simulink model "SAS"  (R2017b)
settings: Solver=VariableStepAuto  StartTime=0.0  StopTime=10.0  RelTol=1e-3
values from neighbouring files (symbols this model uses):
  A = A'    [c_l.m]    (also in c_m.m; c_n.m; c_x.m; c_z.m)
  altitude = input('Enter the altitude for the simulation (ft)  :  ')    [FindF16Dynamics.m]    (also in run_me.m = input(' altitude ( 0 ~ 40000 ft ) : '); trim_F16.m = alt)
  B = ssm_b( state_trim, state_dot_trim, control_trim, xcg )    [ssm_f16.m]    (also in thrust.m = B')
  C = ssm_c( state_trim, state_dot_trim, control_trim, xcg )    [ssm_f16.m]    (also in thrust.m = C')
  C_1 = eye(10)    [run_me.m]
  control_trim = u0    [find_trim.m]
  D = ssm_d( state_trim, state_dot_trim, control_trim, xcg )    [ssm_f16.m]
  D_1 = zeros(10,4)    [run_me.m]
  state_trim = steady_state( state )    [find_trim.m]
  velocity = input('Enter the velocity for the simulation (ft/s):  ')    [FindF16Dynamics.m]    (also in run_me.m = input(' true velocity ( 350 ~ 1000 ft/sec ) : '); trim_F16.m = vel)
libraries: simulink x7
settings Model: Creator=monster  LastModifiedBy=monster

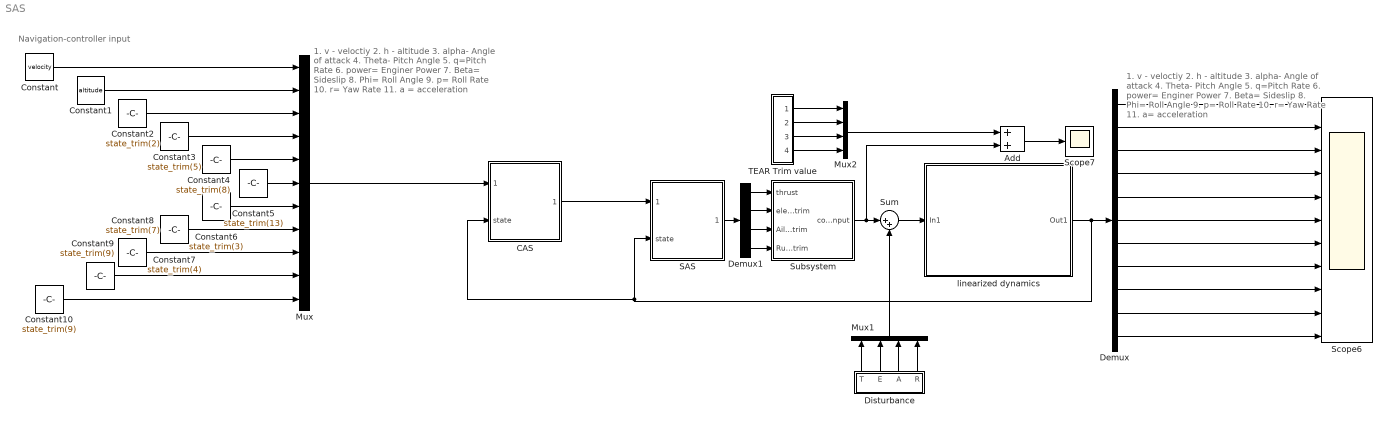
== system SAS ==
  note: Navigation-controller input
  note: 1. v - veloctiy
      |
      | 2. h - altitude
      |
      | 3. alpha- Angle of attack
      |
      | 4. Theta- Pitch Angle
      |
      | 5. q=Pitch Rate
      |
      | 6. power= Enginer Power
      |
      | 7. Beta= Sideslip
      |
      | 8. Phi= Roll Angle
      |
      | 9. p= Roll Rate
      |
      | 10. r= Yaw Rate
      |
      | 11. a= acceleration
  note: 1. v - veloctiy
      |
      | 2. h - altitude
      |
      | 3. alpha- Angle of attack
      |
      | 4. Theta- Pitch Angle
      |
      | 5. q=Pitch Rate
      |
      | 6. power= Enginer Power
      |
      | 7. Beta= Sideslip
      |
      | 8. Phi= Roll Angle
      |
      | 9. p= Roll Rate
      |
      | 10. r= Yaw Rate
      |
      | 11. a = acceleration
  " Disturbance" : Subsystem
  Add : Sum
  CAS : Subsystem
  Constant : Constant  Value=velocity
  Constant1 : Constant  Value=altitude
  Constant10 : Constant  Value=state_trim(9)
  Constant2 : Constant  Value=state_trim(2)
  Constant3 : Constant  Value=state_trim(5)
  Constant4 : Constant  Value=state_trim(8)
  Constant5 : Constant  Value=state_trim(13)
  Constant6 : Constant  Value=state_trim(3)
  Constant7 : Constant  Value=state_trim(4)
  Constant8 : Constant  Value=state_trim(7)
  Constant9 : Constant  Value=state_trim(9)
  Demux : Demux  Outputs=11
  Demux1 : Demux
  Mux : Mux  Inputs=11
  Mux1 : Mux
  Mux2 : Mux
  SAS : Subsystem
  Scope6 : Scope  NumInputPorts=11
  Scope7 : Scope
  Subsystem : Subsystem
  Sum : Sum  Inputs=|++
  "TEAR Trim value " : Subsystem
  linearized dynamics : Subsystem
      mask Display: image('D:\Dropbox\M.eng\fall2017\flight control system\FDC\project\control surface.PNG');
  wires:
  Demux/10 -> Scope6/10
  Subsystem/1(control_input) -> Sum/1, Add/2
  Demux1/1 -> Subsystem/1(thrust)
  Demux1/2 -> Subsystem/2(elevator_trim)
  Demux1/3 -> Subsystem/3(Aileron_trim)
  "TEAR Trim value "/4(R) -> Mux2/4
  Demux/6 -> Scope6/6
  Demux1/4 -> Subsystem/4(Rudder_trim)
  "TEAR Trim value "/1(T) -> Mux2/1
  Demux/7 -> Scope6/7
  "TEAR Trim value "/2(E) -> Mux2/2
  Demux/2 -> Scope6/2
  Add/1 -> Scope7/1
  Demux/4 -> Scope6/4
  Demux/3 -> Scope6/3
  Demux/8 -> Scope6/8
  "TEAR Trim value "/3(A) -> Mux2/3
  Mux2/1 -> Add/1
  Demux/1 -> Scope6/1
  Demux/5 -> Scope6/5
  Demux/9 -> Scope6/9
  SAS/1(control_input) -> Demux1/1
  Mux/1 -> CAS/1(reference)
  Constant7/1 -> Mux/8
  Constant5/1 -> Mux/6
  Constant8/1 -> Mux/9
  Constant9/1 -> Mux/10
  Constant/1 -> Mux/1
  Constant4/1 -> Mux/5
  Constant3/1 -> Mux/4
  Constant2/1 -> Mux/3
  Constant6/1 -> Mux/7
  Constant1/1 -> Mux/2
  linearized dynamics/1(Out1) -> CAS/2(state), SAS/2(state), Demux/1
  Demux/11 -> Scope6/11
  Constant10/1 -> Mux/11
  Sum/1 -> linearized dynamics/1(In1)
  " Disturbance"/4(R) -> Mux1/4
  " Disturbance"/1(T) -> Mux1/1
  " Disturbance"/3(A) -> Mux1/3
  " Disturbance"/2(E) -> Mux1/2
  Mux1/1 -> Sum/2
  CAS/1(control_input) -> SAS/1(reference)

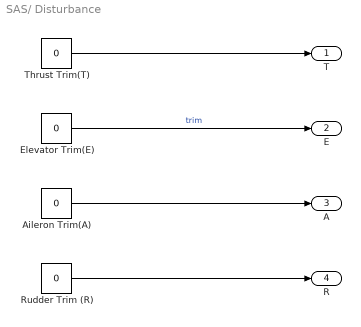
== system SAS/ Disturbance ==
  "Aileron Trim(A) " : Constant  Value=0
  "Elevator Trim(E) " : Constant  Value=0  VectorParams1D=off
  Rudder Trim (R) : Constant  Value=0
  "Thrust Trim(T) " : Constant  Value=0
  T : Outport
  E : Outport  Port=2
  A : Outport  Port=3
  R : Outport  Port=4
  wires:
  "Aileron Trim(A) "/1 -> A/1
  "Elevator Trim(E) "/1 -> E/1  "trim"
  "Thrust Trim(T) "/1 -> T/1
  Rudder Trim (R)/1 -> R/1

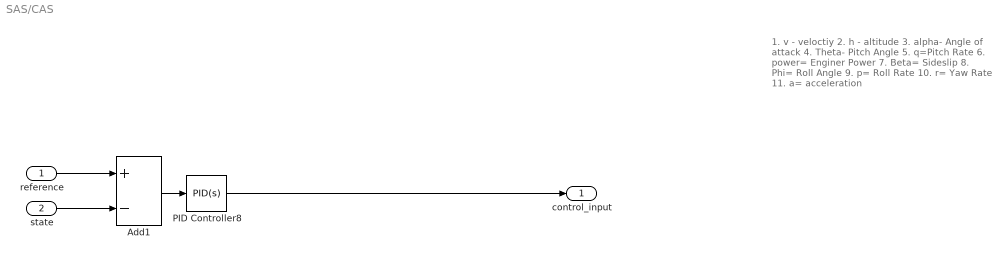
== system SAS/CAS ==
  note: 1. v - veloctiy
      |
      | 2. h - altitude
      |
      | 3. alpha- Angle of attack
      |
      | 4. Theta- Pitch Angle
      |
      | 5. q=Pitch Rate
      |
      | 6. power= Enginer Power
      |
      | 7. Beta= Sideslip
      |
      | 8. Phi= Roll Angle
      |
      | 9. p= Roll Rate
      |
      | 10. r= Yaw Rate
      |
      | 11. a= acceleration
  reference : Inport
  state : Inport  Port=2
  Add1 : Sum  Inputs=+-
  PID Controller8 : simulink/Continuous/PID Controller  Controller=PID  TimeDomain=Continuous-time  SampleTime=-1  IntegratorMethod=Forward Euler  FilterMethod=Forward Euler  Form=Parallel  UseFilter=on  ControllerParametersSource=internal  P=-49327.5398646116  I=-459229.123376859  D=-1288.80480278299  N=1181.77739704053  InitialConditionSource=internal  InitialConditionForIntegrator=0  InitialConditionForFilter=0  ExternalReset=none  LimitOutput=off  UpperSaturationLimit=inf  LowerSaturationLimit=-inf  LinearizeAsGain=on  AntiWindupMode=none  Kb=1  TrackingMode=off  Kt=1  PParamMin=[]  PParamMax=[]  IParamMin=[]  IParamMax=[]  DParamMin=[]  DParamMax=[]  NParamMin=[]  NParamMax=[]  KbParamMin=[]  KbParamMax=[]  KtParamMin=[]  KtParamMax=[]  POutMin=[]  POutMax=[]  IOutMin=[]  IOutMax=[]  DOutMin=[]  DOutMax=[]  NOutMin=[]  NOutMax=[]  KbOutMin=[]  KbOutMax=[]  KtOutMin=[]  KtOutMax=[]  IntegratorOutMin=[]  IntegratorOutMax=[]  FilterOutMin=[]  FilterOutMax=[]  SumOutMin=[]  SumOutMax=[]  SumI1OutMin=[]  SumI1OutMax=[]  SumI2OutMin=[]  SumI2OutMax=[]  SumI3OutMin=[]  SumI3OutMax=[]  SumDOutMin=[]  SumDOutMax=[]  SaturationOutMin=[]  SaturationOutMax=[]  IntegratorContinuousStateAttributes=''  IntegratorStateMustResolveToSignalObject=off  IntegratorRTWStateStorageClass=Auto  FilterContinuousStateAttributes=''  FilterStateMustResolveToSignalObject=off  FilterRTWStateStorageClass=Auto  DifferentiatorICPrevScaledInput=0  DifferentiatorOutMin=[]  DifferentiatorOutMax=[]  InitialConditionSetting=State (most efficient)  FilterDiffOutCoefMin=[]  FilterDiffOutCoefMax=[]  SumDenOutMin=[]  SumDenOutMax=[]  SumNumOutMin=[]  SumNumOutMax=[]  ReciprocalOutMin=[]  ReciprocalOutMax=[]  DivideOutMin=[]  DivideOutMax=[]  TunerSelectOption=Transfer Function Based (PID Tuner App)
  control_input : Outport
  wires:
  PID Controller8/1 -> control_input/1
  Add1/1 -> PID Controller8/1
  reference/1 -> Add1/1
  state/1 -> Add1/2

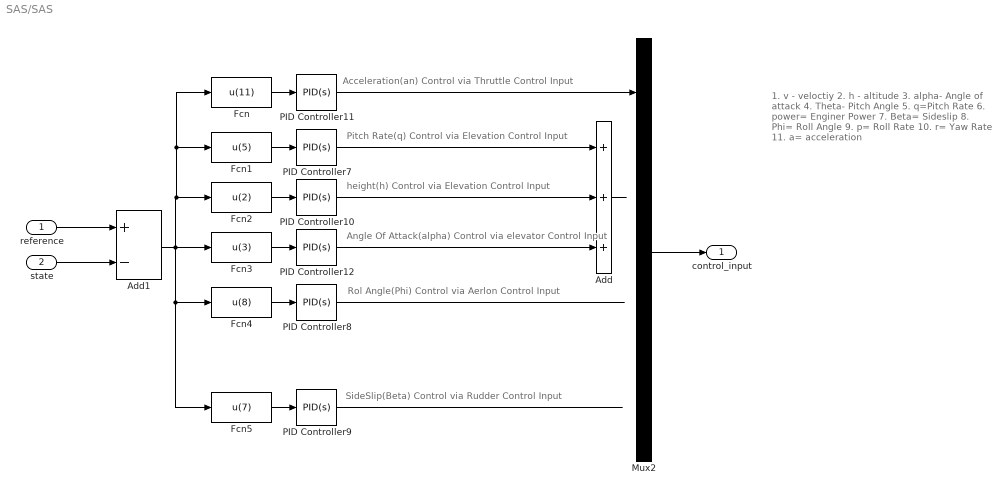
== system SAS/SAS ==
  note: Rol Angle(Phi) Control via Aerlon Control Input
  note: height(h) Control via Elevation Control Input
  note: Pitch Rate(q) Control via Elevation Control Input
  note: Acceleration(an) Control via Thruttle Control Input
  note: Angle Of Attack(alpha) Control via elevator Control Input
  note: SideSlip(Beta) Control via Rudder Control Input
  note: 1. v - veloctiy
      |
      | 2. h - altitude
      |
      | 3. alpha- Angle of attack
      |
      | 4. Theta- Pitch Angle
      |
      | 5. q=Pitch Rate
      |
      | 6. power= Enginer Power
      |
      | 7. Beta= Sideslip
      |
      | 8. Phi= Roll Angle
      |
      | 9. p= Roll Rate
      |
      | 10. r= Yaw Rate
      |
      | 11. a= acceleration
  reference : Inport
  state : Inport  Port=2
  Add : Sum  Inputs=+++
  Add1 : Sum  Inputs=+-
  Fcn : Fcn  Expr=u(11)
  Fcn1 : Fcn  Expr=u(5)
  Fcn2 : Fcn  Expr=u(2)
  Fcn3 : Fcn  Expr=u(3)
  Fcn4 : Fcn  Expr=u(8)
  Fcn5 : Fcn  Expr=u(7)
  Mux2 : Mux
  PID Controller10 : simulink/Continuous/PID Controller  Controller=PID  TimeDomain=Continuous-time  SampleTime=-1  IntegratorMethod=Forward Euler  FilterMethod=Forward Euler  Form=Parallel  UseFilter=on  ControllerParametersSource=internal  P=24508600.1259152  I=4501969741.89748  D=28958.3047379278  N=690409.793644926  InitialConditionSource=internal  InitialConditionForIntegrator=0  InitialConditionForFilter=0  ExternalReset=none  LimitOutput=off  UpperSaturationLimit=inf  LowerSaturationLimit=-inf  LinearizeAsGain=on  AntiWindupMode=none  Kb=1  TrackingMode=off  Kt=1  PParamMin=[]  PParamMax=[]  IParamMin=[]  IParamMax=[]  DParamMin=[]  DParamMax=[]  NParamMin=[]  NParamMax=[]  KbParamMin=[]  KbParamMax=[]  KtParamMin=[]  KtParamMax=[]  POutMin=[]  POutMax=[]  IOutMin=[]  IOutMax=[]  DOutMin=[]  DOutMax=[]  NOutMin=[]  NOutMax=[]  KbOutMin=[]  KbOutMax=[]  KtOutMin=[]  KtOutMax=[]  IntegratorOutMin=[]  IntegratorOutMax=[]  FilterOutMin=[]  FilterOutMax=[]  SumOutMin=[]  SumOutMax=[]  SumI1OutMin=[]  SumI1OutMax=[]  SumI2OutMin=[]  SumI2OutMax=[]  SumI3OutMin=[]  SumI3OutMax=[]  SumDOutMin=[]  SumDOutMax=[]  SaturationOutMin=[]  SaturationOutMax=[]  IntegratorContinuousStateAttributes=''  IntegratorStateMustResolveToSignalObject=off  IntegratorRTWStateStorageClass=Auto  FilterContinuousStateAttributes=''  FilterStateMustResolveToSignalObject=off  FilterRTWStateStorageClass=Auto  DifferentiatorICPrevScaledInput=0  DifferentiatorOutMin=[]  DifferentiatorOutMax=[]  InitialConditionSetting=State (most efficient)  FilterDiffOutCoefMin=[]  FilterDiffOutCoefMax=[]  SumDenOutMin=[]  SumDenOutMax=[]  SumNumOutMin=[]  SumNumOutMax=[]  ReciprocalOutMin=[]  ReciprocalOutMax=[]  DivideOutMin=[]  DivideOutMax=[]  TunerSelectOption=Transfer Function Based (PID Tuner App)
  PID Controller11 : simulink/Continuous/PID Controller  Controller=PID  TimeDomain=Continuous-time  SampleTime=-1  IntegratorMethod=Forward Euler  FilterMethod=Forward Euler  Form=Parallel  UseFilter=on  ControllerParametersSource=internal  P=13329483.1324469  I=392847306.175743  D=98980.5300334758  N=109037.560099343  InitialConditionSource=internal  InitialConditionForIntegrator=0  InitialConditionForFilter=0  ExternalReset=none  LimitOutput=off  UpperSaturationLimit=inf  LowerSaturationLimit=-inf  LinearizeAsGain=on  AntiWindupMode=none  Kb=1  TrackingMode=off  Kt=1  PParamMin=[]  PParamMax=[]  IParamMin=[]  IParamMax=[]  DParamMin=[]  DParamMax=[]  NParamMin=[]  NParamMax=[]  KbParamMin=[]  KbParamMax=[]  KtParamMin=[]  KtParamMax=[]  POutMin=[]  POutMax=[]  IOutMin=[]  IOutMax=[]  DOutMin=[]  DOutMax=[]  NOutMin=[]  NOutMax=[]  KbOutMin=[]  KbOutMax=[]  KtOutMin=[]  KtOutMax=[]  IntegratorOutMin=[]  IntegratorOutMax=[]  FilterOutMin=[]  FilterOutMax=[]  SumOutMin=[]  SumOutMax=[]  SumI1OutMin=[]  SumI1OutMax=[]  SumI2OutMin=[]  SumI2OutMax=[]  SumI3OutMin=[]  SumI3OutMax=[]  SumDOutMin=[]  SumDOutMax=[]  SaturationOutMin=[]  SaturationOutMax=[]  IntegratorContinuousStateAttributes=''  IntegratorStateMustResolveToSignalObject=off  IntegratorRTWStateStorageClass=Auto  FilterContinuousStateAttributes=''  FilterStateMustResolveToSignalObject=off  FilterRTWStateStorageClass=Auto  DifferentiatorICPrevScaledInput=0  DifferentiatorOutMin=[]  DifferentiatorOutMax=[]  InitialConditionSetting=State (most efficient)  FilterDiffOutCoefMin=[]  FilterDiffOutCoefMax=[]  SumDenOutMin=[]  SumDenOutMax=[]  SumNumOutMin=[]  SumNumOutMax=[]  ReciprocalOutMin=[]  ReciprocalOutMax=[]  DivideOutMin=[]  DivideOutMax=[]  TunerSelectOption=Transfer Function Based (PID Tuner App)
  PID Controller12 : simulink/Continuous/PID Controller  Controller=PID  TimeDomain=Continuous-time  SampleTime=-1  IntegratorMethod=Forward Euler  FilterMethod=Forward Euler  Form=Parallel  UseFilter=on  ControllerParametersSource=internal  P=-170.14183467408  I=-465.695324804371  D=-13.6839697818054  N=105.697856042613  InitialConditionSource=internal  InitialConditionForIntegrator=0  InitialConditionForFilter=0  ExternalReset=none  LimitOutput=off  UpperSaturationLimit=inf  LowerSaturationLimit=-inf  LinearizeAsGain=on  AntiWindupMode=none  Kb=1  TrackingMode=off  Kt=1  PParamMin=[]  PParamMax=[]  IParamMin=[]  IParamMax=[]  DParamMin=[]  DParamMax=[]  NParamMin=[]  NParamMax=[]  KbParamMin=[]  KbParamMax=[]  KtParamMin=[]  KtParamMax=[]  POutMin=[]  POutMax=[]  IOutMin=[]  IOutMax=[]  DOutMin=[]  DOutMax=[]  NOutMin=[]  NOutMax=[]  KbOutMin=[]  KbOutMax=[]  KtOutMin=[]  KtOutMax=[]  IntegratorOutMin=[]  IntegratorOutMax=[]  FilterOutMin=[]  FilterOutMax=[]  SumOutMin=[]  SumOutMax=[]  SumI1OutMin=[]  SumI1OutMax=[]  SumI2OutMin=[]  SumI2OutMax=[]  SumI3OutMin=[]  SumI3OutMax=[]  SumDOutMin=[]  SumDOutMax=[]  SaturationOutMin=[]  SaturationOutMax=[]  IntegratorContinuousStateAttributes=''  IntegratorStateMustResolveToSignalObject=off  IntegratorRTWStateStorageClass=Auto  FilterContinuousStateAttributes=''  FilterStateMustResolveToSignalObject=off  FilterRTWStateStorageClass=Auto  DifferentiatorICPrevScaledInput=0  DifferentiatorOutMin=[]  DifferentiatorOutMax=[]  InitialConditionSetting=State (most efficient)  FilterDiffOutCoefMin=[]  FilterDiffOutCoefMax=[]  SumDenOutMin=[]  SumDenOutMax=[]  SumNumOutMin=[]  SumNumOutMax=[]  ReciprocalOutMin=[]  ReciprocalOutMax=[]  DivideOutMin=[]  DivideOutMax=[]  TunerSelectOption=Transfer Function Based (PID Tuner App)
  PID Controller7 : simulink/Continuous/PID Controller  Controller=PID  TimeDomain=Continuous-time  SampleTime=-1  IntegratorMethod=Forward Euler  FilterMethod=Forward Euler  Form=Parallel  UseFilter=on  ControllerParametersSource=internal  P=-2409.99420452658  I=-41171.6281036838  D=-4.63151383685818  N=352.425457454863  InitialConditionSource=internal  InitialConditionForIntegrator=0  InitialConditionForFilter=0  ExternalReset=none  LimitOutput=off  UpperSaturationLimit=inf  LowerSaturationLimit=-inf  LinearizeAsGain=on  AntiWindupMode=none  Kb=1  TrackingMode=off  Kt=1  PParamMin=[]  PParamMax=[]  IParamMin=[]  IParamMax=[]  DParamMin=[]  DParamMax=[]  NParamMin=[]  NParamMax=[]  KbParamMin=[]  KbParamMax=[]  KtParamMin=[]  KtParamMax=[]  POutMin=[]  POutMax=[]  IOutMin=[]  IOutMax=[]  DOutMin=[]  DOutMax=[]  NOutMin=[]  NOutMax=[]  KbOutMin=[]  KbOutMax=[]  KtOutMin=[]  KtOutMax=[]  IntegratorOutMin=[]  IntegratorOutMax=[]  FilterOutMin=[]  FilterOutMax=[]  SumOutMin=[]  SumOutMax=[]  SumI1OutMin=[]  SumI1OutMax=[]  SumI2OutMin=[]  SumI2OutMax=[]  SumI3OutMin=[]  SumI3OutMax=[]  SumDOutMin=[]  SumDOutMax=[]  SaturationOutMin=[]  SaturationOutMax=[]  IntegratorContinuousStateAttributes=''  IntegratorStateMustResolveToSignalObject=off  IntegratorRTWStateStorageClass=Auto  FilterContinuousStateAttributes=''  FilterStateMustResolveToSignalObject=off  FilterRTWStateStorageClass=Auto  DifferentiatorICPrevScaledInput=0  DifferentiatorOutMin=[]  DifferentiatorOutMax=[]  InitialConditionSetting=State (most efficient)  FilterDiffOutCoefMin=[]  FilterDiffOutCoefMax=[]  SumDenOutMin=[]  SumDenOutMax=[]  SumNumOutMin=[]  SumNumOutMax=[]  ReciprocalOutMin=[]  ReciprocalOutMax=[]  DivideOutMin=[]  DivideOutMax=[]  TunerSelectOption=Transfer Function Based (PID Tuner App)
  PID Controller8 : simulink/Continuous/PID Controller  Controller=PID  TimeDomain=Continuous-time  SampleTime=-1  IntegratorMethod=Forward Euler  FilterMethod=Forward Euler  Form=Parallel  UseFilter=on  ControllerParametersSource=internal  P=-49327.5398646116  I=-459229.123376859  D=-1288.80480278299  N=1181.77739704053  InitialConditionSource=internal  InitialConditionForIntegrator=0  InitialConditionForFilter=0  ExternalReset=none  LimitOutput=off  UpperSaturationLimit=inf  LowerSaturationLimit=-inf  LinearizeAsGain=on  AntiWindupMode=none  Kb=1  TrackingMode=off  Kt=1  PParamMin=[]  PParamMax=[]  IParamMin=[]  IParamMax=[]  DParamMin=[]  DParamMax=[]  NParamMin=[]  NParamMax=[]  KbParamMin=[]  KbParamMax=[]  KtParamMin=[]  KtParamMax=[]  POutMin=[]  POutMax=[]  IOutMin=[]  IOutMax=[]  DOutMin=[]  DOutMax=[]  NOutMin=[]  NOutMax=[]  KbOutMin=[]  KbOutMax=[]  KtOutMin=[]  KtOutMax=[]  IntegratorOutMin=[]  IntegratorOutMax=[]  FilterOutMin=[]  FilterOutMax=[]  SumOutMin=[]  SumOutMax=[]  SumI1OutMin=[]  SumI1OutMax=[]  SumI2OutMin=[]  SumI2OutMax=[]  SumI3OutMin=[]  SumI3OutMax=[]  SumDOutMin=[]  SumDOutMax=[]  SaturationOutMin=[]  SaturationOutMax=[]  IntegratorContinuousStateAttributes=''  IntegratorStateMustResolveToSignalObject=off  IntegratorRTWStateStorageClass=Auto  FilterContinuousStateAttributes=''  FilterStateMustResolveToSignalObject=off  FilterRTWStateStorageClass=Auto  DifferentiatorICPrevScaledInput=0  DifferentiatorOutMin=[]  DifferentiatorOutMax=[]  InitialConditionSetting=State (most efficient)  FilterDiffOutCoefMin=[]  FilterDiffOutCoefMax=[]  SumDenOutMin=[]  SumDenOutMax=[]  SumNumOutMin=[]  SumNumOutMax=[]  ReciprocalOutMin=[]  ReciprocalOutMax=[]  DivideOutMin=[]  DivideOutMax=[]  TunerSelectOption=Transfer Function Based (PID Tuner App)
  PID Controller9 : simulink/Continuous/PID Controller  Controller=PID  TimeDomain=Continuous-time  SampleTime=-1  IntegratorMethod=Forward Euler  FilterMethod=Forward Euler  Form=Parallel  UseFilter=on  ControllerParametersSource=internal  P=908.491475757153  I=143.160579860217  D=1280.97081759687  N=3086.89831654681  InitialConditionSource=internal  InitialConditionForIntegrator=0  InitialConditionForFilter=0  ExternalReset=none  LimitOutput=off  UpperSaturationLimit=inf  LowerSaturationLimit=-inf  LinearizeAsGain=on  AntiWindupMode=none  Kb=1  TrackingMode=off  Kt=1  PParamMin=[]  PParamMax=[]  IParamMin=[]  IParamMax=[]  DParamMin=[]  DParamMax=[]  NParamMin=[]  NParamMax=[]  KbParamMin=[]  KbParamMax=[]  KtParamMin=[]  KtParamMax=[]  POutMin=[]  POutMax=[]  IOutMin=[]  IOutMax=[]  DOutMin=[]  DOutMax=[]  NOutMin=[]  NOutMax=[]  KbOutMin=[]  KbOutMax=[]  KtOutMin=[]  KtOutMax=[]  IntegratorOutMin=[]  IntegratorOutMax=[]  FilterOutMin=[]  FilterOutMax=[]  SumOutMin=[]  SumOutMax=[]  SumI1OutMin=[]  SumI1OutMax=[]  SumI2OutMin=[]  SumI2OutMax=[]  SumI3OutMin=[]  SumI3OutMax=[]  SumDOutMin=[]  SumDOutMax=[]  SaturationOutMin=[]  SaturationOutMax=[]  IntegratorContinuousStateAttributes=''  IntegratorStateMustResolveToSignalObject=off  IntegratorRTWStateStorageClass=Auto  FilterContinuousStateAttributes=''  FilterStateMustResolveToSignalObject=off  FilterRTWStateStorageClass=Auto  DifferentiatorICPrevScaledInput=0  DifferentiatorOutMin=[]  DifferentiatorOutMax=[]  InitialConditionSetting=State (most efficient)  FilterDiffOutCoefMin=[]  FilterDiffOutCoefMax=[]  SumDenOutMin=[]  SumDenOutMax=[]  SumNumOutMin=[]  SumNumOutMax=[]  ReciprocalOutMin=[]  ReciprocalOutMax=[]  DivideOutMin=[]  DivideOutMax=[]  TunerSelectOption=Transfer Function Based (PID Tuner App)
  control_input : Outport
  wires:
  Mux2/1 -> control_input/1
  PID Controller11/1 -> Mux2/1
  Fcn5/1 -> PID Controller9/1
  Fcn3/1 -> PID Controller12/1
  PID Controller7/1 -> Add/1
  Fcn2/1 -> PID Controller10/1
  Fcn1/1 -> PID Controller7/1
  PID Controller8/1 -> ?
  Fcn4/1 -> PID Controller8/1
  Fcn/1 -> PID Controller11/1
  PID Controller10/1 -> Add/2
  Add/1 -> ?
  PID Controller12/1 -> Add/3
  PID Controller9/1 -> ?
  reference/1 -> Add1/1
  state/1 -> Add1/2
  Add1/1 -> Fcn2/1, Fcn1/1, Fcn/1, Fcn5/1, Fcn4/1, Fcn3/1

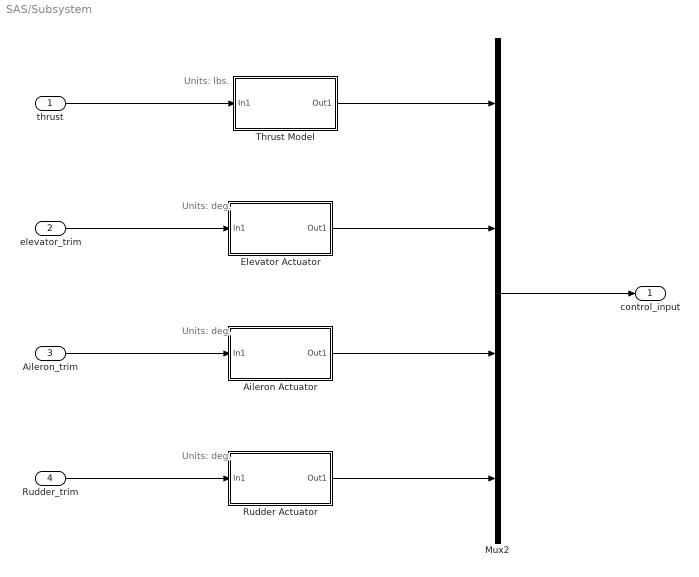
== system SAS/Subsystem ==
  note: Units: deg.
  note: Units: deg.
  note: Units: lbs.
  note: Units: deg.
  thrust : Inport
  elevator_trim : Inport  Port=2
  Aileron_trim : Inport  Port=3
  Rudder_trim : Inport  Port=4
  Aileron Actuator : Subsystem  AncestorBlock=F16_Actuator_Library/Aileron Actuator
  Elevator Actuator : Subsystem  AncestorBlock=F16_Actuator_Library/Elevator Actuator
  Mux2 : Mux
  Rudder Actuator : Subsystem  AncestorBlock=F16_Actuator_Library/Rudder Actuator
  Thrust Model : Subsystem  AncestorBlock=F16_Actuator_Library/Thrust Model
  control_input : Outport
  wires:
  thrust/1 -> Thrust Model/1(In1)
  Aileron Actuator/1(Out1) -> Mux2/3
  Rudder_trim/1 -> Rudder Actuator/1(In1)
  Elevator Actuator/1(Out1) -> Mux2/2
  Rudder Actuator/1(Out1) -> Mux2/4
  elevator_trim/1 -> Elevator Actuator/1(In1)
  Aileron_trim/1 -> Aileron Actuator/1(In1)
  Thrust Model/1(Out1) -> Mux2/1
  Mux2/1 -> control_input/1

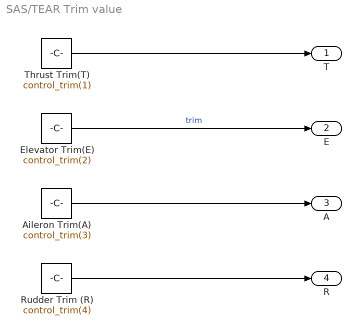
== system SAS/TEAR Trim value  ==
  "Aileron Trim(A) " : Constant  Value=control_trim(3)
  "Elevator Trim(E) " : Constant  Value=control_trim(2)  VectorParams1D=off
  Rudder Trim (R) : Constant  Value=control_trim(4)
  "Thrust Trim(T) " : Constant  Value=control_trim(1)
  T : Outport
  E : Outport  Port=2
  A : Outport  Port=3
  R : Outport  Port=4
  wires:
  "Aileron Trim(A) "/1 -> A/1
  "Elevator Trim(E) "/1 -> E/1  "trim"
  "Thrust Trim(T) "/1 -> T/1
  Rudder Trim (R)/1 -> R/1

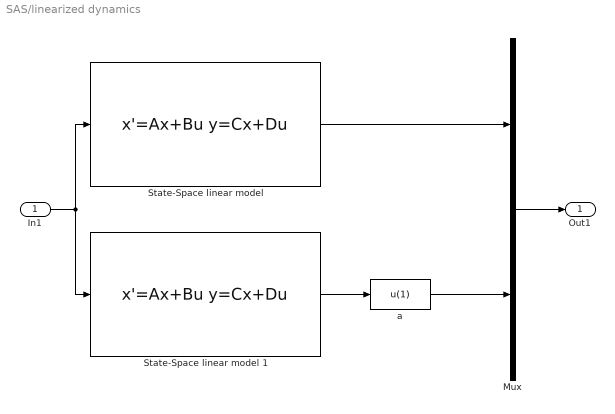
== system SAS/linearized dynamics ==
  In1 : Inport
  Mux : Mux  Inputs=2
  "State-Space linear model " : StateSpace  A=A  B=B  C=C_1  D=D_1  InitialCondition=[state_trim(1);state_trim(12);state_trim(2);state_trim(5);state_trim(8);state_trim(13);state_trim(3);state_trim(4);state_trim(7);state_trim(9)]
      mask Display: image('D:\Dropbox\M.eng\fall2017\flight control system\FDC\project\control surface.PNG');
  State-Space linear model 1 : StateSpace  A=A  B=B  C=C  D=D  InitialCondition=[state_trim(1);state_trim(12);state_trim(2);state_trim(5);state_trim(8);state_trim(13);state_trim(3);state_trim(4);state_trim(7);state_trim(9)]
      mask Display: image('D:\Dropbox\M.eng\fall2017\flight control system\FDC\project\control surface.PNG');
  a : Fcn  Expr=u(1)
  Out1 : Outport
  wires:
  a/1 -> Mux/2
  In1/1 -> "State-Space linear model "/1, State-Space linear model 1/1
  "State-Space linear model "/1 -> Mux/1
  State-Space linear model 1/1 -> a/1
  Mux/1 -> Out1/1

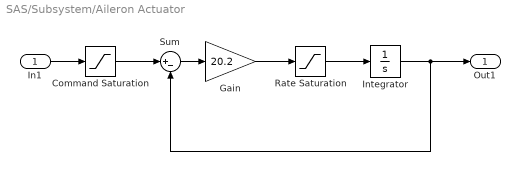
== system SAS/Subsystem/Aileron Actuator ==
  In1 : Inport
  Command Saturation : Saturate  UpperLimit=21.5  LowerLimit=-21.5
  Gain : Gain  Gain=20.2  SaturateOnIntegerOverflow=on  OutDataTypeStr=Inherit: Same as input  ParamDataTypeStr=Inherit: Same as input
  "Integrator " : Integrator  InitialCondition=control_trim(2)  UpperSaturationLimit=21.5  LowerSaturationLimit=-21.5
  Rate Saturation : Saturate  UpperLimit=80  LowerLimit=-80
  Sum : Sum  Inputs=|+-  SaturateOnIntegerOverflow=on  InputSameDT=on  OutDataTypeStr=Inherit: Same as first input
  Out1 : Outport
  wires:
  "Integrator "/1 -> Sum/2, Out1/1
  Rate Saturation/1 -> "Integrator "/1
  Gain/1 -> Rate Saturation/1
  Sum/1 -> Gain/1
  Command Saturation/1 -> Sum/1
  In1/1 -> Command Saturation/1

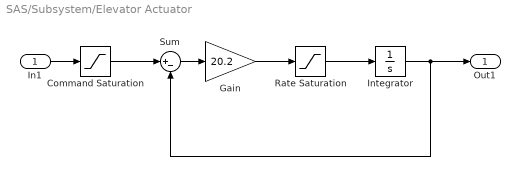
== system SAS/Subsystem/Elevator Actuator ==
  In1 : Inport
  Command Saturation : Saturate  UpperLimit=25  LowerLimit=-25
  Gain : Gain  Gain=20.2  SaturateOnIntegerOverflow=on  OutDataTypeStr=Inherit: Same as input  ParamDataTypeStr=Inherit: Same as input
  "Integrator " : Integrator  InitialCondition=control_trim(2)  UpperSaturationLimit=25  LowerSaturationLimit=-25
  Rate Saturation : Saturate  UpperLimit=60  LowerLimit=-60
  Sum : Sum  Inputs=|+-  SaturateOnIntegerOverflow=on  InputSameDT=on  OutDataTypeStr=Inherit: Same as first input
  Out1 : Outport
  wires:
  "Integrator "/1 -> Sum/2, Out1/1
  Rate Saturation/1 -> "Integrator "/1
  Gain/1 -> Rate Saturation/1
  Sum/1 -> Gain/1
  Command Saturation/1 -> Sum/1
  In1/1 -> Command Saturation/1

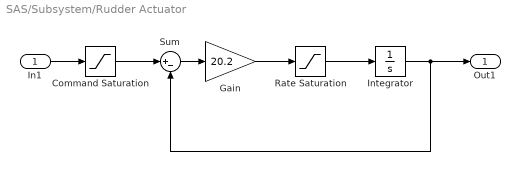
== system SAS/Subsystem/Rudder Actuator ==
  In1 : Inport
  Command Saturation : Saturate  UpperLimit=30  LowerLimit=-30
  Gain : Gain  Gain=20.2  SaturateOnIntegerOverflow=on  OutDataTypeStr=Inherit: Same as input  ParamDataTypeStr=Inherit: Same as input
  "Integrator " : Integrator  InitialCondition=control_trim(2)  UpperSaturationLimit=30  LowerSaturationLimit=-30
  Rate Saturation : Saturate  UpperLimit=120  LowerLimit=-120
  Sum : Sum  Inputs=|+-  SaturateOnIntegerOverflow=on  InputSameDT=on  OutDataTypeStr=Inherit: Same as first input
  Out1 : Outport
  wires:
  "Integrator "/1 -> Sum/2, Out1/1
  Rate Saturation/1 -> "Integrator "/1
  Gain/1 -> Rate Saturation/1
  Sum/1 -> Gain/1
  Command Saturation/1 -> Sum/1
  In1/1 -> Command Saturation/1

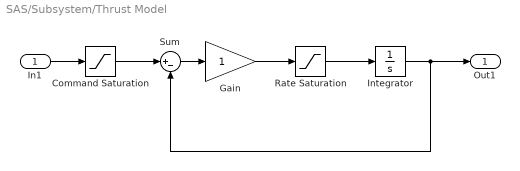
== system SAS/Subsystem/Thrust Model ==
  In1 : Inport
  Command Saturation : Saturate  UpperLimit=19000  LowerLimit=1000
  Gain : Gain  SaturateOnIntegerOverflow=on  OutDataTypeStr=Inherit: Same as input  ParamDataTypeStr=Inherit: Same as input
  "Integrator " : Integrator  InitialCondition=control_trim(1)  UpperSaturationLimit=30  LowerSaturationLimit=-30
  Rate Saturation : Saturate  UpperLimit=10000  LowerLimit=-10000
  Sum : Sum  Inputs=|+-  SaturateOnIntegerOverflow=on  InputSameDT=on  OutDataTypeStr=Inherit: Same as first input
  Out1 : Outport
  wires:
  "Integrator "/1 -> Sum/2, Out1/1
  Rate Saturation/1 -> "Integrator "/1
  Gain/1 -> Rate Saturation/1
  Sum/1 -> Gain/1
  Command Saturation/1 -> Sum/1
  In1/1 -> Command Saturation/1
